simulink model "five_bar_model_discrete_v_0"  (R2018a)
settings: Solver=ode45  StartTime=0.0  StopTime=tmax  FixedStep=0.0001  MaxStep=1e-3  RelTol=1e-3
values from neighbouring files (symbols this model uses):
  dt = 10e-3    (= 0.01)    [model_parameters_v_1.m]    (also in test_dynamics.m = 0.2; test_kinematics.m = 0.1)
  g = -9.80665    [idyn5.m]    (also in test_dynamics.m; test_model.m = 9.80665)
  Kd = (3*aj*wj-Fv) * eye(2)    [model_parameters_v_1.m]
  Kdi = [2 * zita *  wpos1; 2  * zita * wpos2]    [model_parameters_v_1.m]
  Ki = aj*wj^3 * eye(2)    [model_parameters_v_1.m]
  Kp = 3*aj*wj^2 * eye(2)    [model_parameters_v_1.m]
  Kpi = [ wpos1^2;  wpos2^2]    [model_parameters_v_1.m]
  p = [NaN; NaN]    [fkine5.m]    (also in test_model.m = zeros(n,2))
  p0 = p(:,1)    [model_parameters_v_1.m]    (also in test_dynamics.m = [x(i);y(i)]; test_kinematics.m = [0; 0.35])
  q = [NaN; NaN; NaN; NaN; NaN]    [fkine5.m]    (also in ikine5.m = [q11;q12;q13;q21;q22])
  q0 = q(:,1)    [model_parameters_v_1.m]    (also in test_dynamics.m = q0(:,4); test_kinematics.m = q0(:,4))
  qd = [qda(1);qdu(1);qdu(2);qda(2);qdu(3)]    [ifirstkine5.m]
  qdd = [qdda(1);qddu(1);qddu(2);qdda(2);qddu(3)]    [isecondkine5.m]
  t0r = J * qda    [ffirstkine5.m]    (also in test_dynamics.m = [0;0]; test_kinematics.m = [1;1]; test_model.m = p)
  t0r0 = t0r(:,1)    [model_parameters_v_1.m]
  t0rd = (J * qdda+ at)    [fsecondkine5.m]    (also in test_dynamics.m = [0;0]; test_kinematics.m = [-1;1]; test_model.m = p)
  t0rd0 = t0rd(:,1)    [model_parameters_v_1.m]
undefined symbols (not defined in the file or in its folder): DiscIntNeverNeededParam, Kii, tmax, X, Y, Z
libraries: sm_lib x24, simulink x16, nesl_utility x9, powerlib_meascontrol x1
(part 3 of 3)

== matlab function five_bar_model_discrete_v_0/five-bar-robot2/forward kinematics ==
  data: qa input; p output; assembly input; q output
function [p,q] = fkine5(qa, assembly)
% This function implement the forward kinematic model of a five bar robot
% @parm qa: active joint positions vector 2x1
% @parm assembly: assembly mode selecction 1 for + -1 for -
% @return p: p end-effector coordinate vector 2X1
% @return q: joint positon vector 5X1
    l = 0.205;
    d1 = [-0.125, l, l];
    d2 = [0.125, l, l];
    q11 = qa(1);
    q21 = qa(2);

    A12 = [d1(2)*cos(q11)+d1(1); d1(2)*sin(q11)];
    A22 = [d2(2)*cos(q21)+d2(1); d2(2)*sin(q21)];

    if sqrt((A12-A22)' * (A12-A22)) <= 2*l
        a1 = - 2*d1(1) - 2*d1(2)*cos(q11);
        a2 = - 2*d2(1) - 2*d2(2)*cos(q21);
        b1 = - 2*sin(q11)*d1(2);
        b2 = - 2*sin(q21)*d2(2);
        c1 = d1(1)^2 + 2*cos(q11)*d1(1)*d1(2) + d1(2)^2 - d1(3)^2;
        c2 = d2(1)^2 + 2*cos(q21)*d2(1)*d2(2) + d2(2)^2 - d2(3)^2;

        if b1 ~= b2
            a = a2 - a1;
            b = b2 - b1;
            c = c2 - c1;
            e1 = - a / b;
            e2 = - c / b;
            f1 = 1 + e1^2;
            f2 = 2 * e1 * e2 + a1 + b1 * e1;
            f3 = e2^2 + b1 * e2 + c1;

            x = (-f2 - sqrt(f2^2 - 4 * f1 * f3)) / (2 * f1);
            y = e1 * x + e2;

            A13=[x-A12(1);y-A12(2)];
            A23=[x-A22(1);y-A22(2)];
            if  A13(1)*A23(2)-A23(1)*A13(2) <= 0 && assembly == 1
                x = (-f2 + sqrt(f2^2 - 4 * f1 * f3)) / (2 * f1);
                y = e1 * x + e2;
            elseif  A13(1)*A23(2)-A23(1)*A13(2) >= 0 && assembly == -1
                x = (-f2 + sqrt(f2^2 - 4 * f1 * f3)) / (2 * f1);
                y = e1 * x + e2;
            end
        else
            x = - (c2 - c1) / (a2 - a1);
            y = (-b1 + (b1^2 - 4 * (x^2 + a1 * x + c1))^(1/2)) / 2;

            A13=[x-A12(1);y-A12(2)];
            A23=[x-A22(1);y-A22(2)];
            if  A13(1)*A23(2)-A23(1)*A13(2) <= 0 && assembly == 1
                y = (-b1 - (b1^2 - 4 * (x^2 + a1 * x + c1))^(1/2)) / 2;
            elseif  A13(1)*A23(2)-A23(1)*A13(2) >= 0 && assembly == -1
                y = (-b1 - (b1^2 - 4 * (x^2 + a1 * x + c1))^(1/2)) / 2;
            end
        end

        % for q12 and q22 from a12/a11 and a22/a21
        q12 = atan2(y-d1(2)*sin(q11), x-d1(1)-d1(2)*cos(q11)) - q11;
        q22 = atan2(y-d2(2)*sin(q21), x-d2(1)-d2(2)*cos(q21)) - q21;
        q13 = q21 + q22 - q11 - q12;
        p = [x;y];
        q = [q11; q12; q13; q21; q22];
        
        % I will work in the first assembly.
        % Note: A way of implement the change of assembly is using the equations
        % (3) and (4) of the paper Minimum-time trajectory planning and control
        % of a pick-and-place five-bar parallel robot. Obtaining the
        % previous assembly, then the current and finally comparing
        % eache other.
%         sum(angdiff(q, q_prev).^2)
%         if sum(angdiff(q, q_prev).^2) > 0.1 
%             disp('Atention!!');
%             assembly2 = -assembly;
%             q11 = qa(1);
%             q21 = qa(2);
%             a1 = - 2*d1(1) - 2*d1(2)*cos(q11);
%             a2 = - 2*d2(1) - 2*d2(2)*cos(q21);
%             b1 = - 2*sin(q11)*d1(2);
%             b2 = - 2*sin(q21)*d2(2);
%             c1 = d1(1)^2 + 2*cos(q11)*d1(1)*d1(2) + d1(2)^2 - d1(3)^2;
%             c2 = d2(1)^2 + 2*cos(q21)*d2(1)*d2(2) + d2(2)^2 - d2(3)^2;
% 
%             if b1 ~= b2
%                 a = a2 - a1;
%                 b = b2 - b1;
%                 c = c2 - c1;
%                 e1 = - a / b;
%                 e2 = - c / b;
%                 f1 = 1 + e1^2;
%                 f2 = 2 * e1 * e2 + a1 + b1 * e1;
%                 f3 = e2^2 + b1 * e2 + c1;
% 
%                 x = (-f2 - sqrt(f2^2 - 4 * f1 * f3)) / (2 * f1);
%                 y = e1 * x + e2;
% 
%                 A13=[x-A12(1);y-A12(2)];
%                 A23=[x-A22(1);y-A22(2)];
%                 if  A13(1)*A23(2)-A23(1)*A13(2) <= 0 && assembly2 == 1
%                     x = (-f2 + sqrt(f2^2 - 4 * f1 * f3)) / (2 * f1);
%                     y = e1 * x + e2;
%                 elseif  A13(1)*A23(2)-A23(1)*A13(2) >= 0 && assembly2 == -1
%                     x = (-f2 + sqrt(f2^2 - 4 * f1 * f3)) / (2 * f1);
%                     y = e1 * x + e2;
%                 end
%             else
%                 x = - (c2 - c1) / (a2 - a1);
%                 y = (-b1 + (b1^2 - 4 * (x^2 + a1 * x + c1))^(1/2)) / 2;
% 
%                 A13=[x-A12(1);y-A12(2)];
%                 A23=[x-A22(1);y-A22(2)];
%                 if  A13(1)*A23(2)-A23(1)*A13(2) <= 0 && assembly == 1
%                     y = (-b1 - (b1^2 - 4 * (x^2 + a1 * x + c1))^(1/2)) / 2;
%                 elseif  A13(1)*A23(2)-A23(1)*A13(2) >= 0 && assembly == -1
%                     y = (-b1 - (b1^2 - 4 * (x^2 + a1 * x + c1))^(1/2)) / 2;
%                 end
%             end
% 
%             % for q12 and q22 from a12/a11 and a22/a21
%             q12 = atan2(y-d1(2)*sin(q11), x-d1(1)-d1(2)*cos(q11)) - q11;
%             q22 = atan2(y-d2(2)*sin(q21), x-d2(1)-d2(2)*cos(q21)) - q21;
%             q13 = q21 + q22 - q11 - q12;
%             p = [x;y];
%             q = [q11; q12; q13; q21; q22];
%         end
    else
        disp('ERROR: Euclidian distance > 2*l');
        p = [NaN; NaN];
        q = [NaN; NaN; NaN; NaN; NaN];
    end

== matlab function five_bar_model_discrete_v_0/five-bar-robot2/inverse dynamics ==
  data: q input; T output double size=2; qd input; qdd input; t0rd input; J input; Jt input; Jta input; Jtd input; Psit input
function T  = idyn5(q,qd,qdd,t0rd,J,Jt,Jta,Jtd,Psit)

    l = 0.205;
    d1 = [-0.125, l, l];
    d2 = [0.125, l, l];
    q1 = q(1:3);
    q2 = q(4:5);
    qd1 = qd(1:3);
    qd2 = qd(4:5);
    qdd1 = qdd(1:3);
    qdd2 = qdd(4:5);
    xdd = t0rd(1);
    ydd = t0rd(2);
    Tt1 = zeros(3,1);
    Tt2 = zeros(2,1);
    Ttd = zeros(3,1);
    % Dynamic
    % Gravity 
%     g = -9.80665;
    g = 0;
% Dynamics parameters
    m11 = 0.126; %kg
    mx11 = m11 * 0.1025;
    my11 =  0; %m11 * 1.44e-2;
    zz11 = 0.001774; %kg-m^2;
    
    m12 = 0.126; %kg
    mx12 = m12 * 0.1025;
    my12 =  0; %m11 * 1.44e-2;
    zz12 = 0.001774; %kg-m^2;
    
    m21 = 0.126; %kg
    mx21 = m21 * 0.1025;
    my21 =  0; %m11 * 1.44e-2;
    zz21 = 0.001774; %kg-m^2;
    
    m22 = 0.126; %kg
    mx22 = m22 * 0.1025;
    my22 =  0; %m11 * 1.44e-2;
    zz22 = 0.001774; %kg-m^2;
    
    Ia11 = 4.8e-5; % kg-m2
%     zz11r = zz11 + Ia11 + d1(2)^2 * m12;
    
    Ia21 = 4.8e-5; % kg-m2
%     zz21r = zz21 + Ia21 + d2(2)^2 * m22;
   
    %Fricciones fv = viscosa fs= seca
    fv1 = [1.5e-1 0 0];
    fs1 = [1.5e-1 0 0];
    fv2 = [0 0];
    fs2 = [0 0];
    % End effector mass
    m4 = 0.272;

    % Inverse dynamics model
    Tt1(1) = (my12*sin(q1(1) + q1(2)) - mx12*cos(q1(1) + q1(2)) ...
        - mx11*cos(q1(1)) + my11*sin(q1(1)) - d1(2)*m12*cos(q1(1)))*g ...
        + Ia11*qdd1(1) + fv1(1)*qd1(1) + fs1(1)*sign(qd1(1)) ...
        + mx12*(- d1(2)*sin(q1(2))*qd1(2)^2 - 2*d1(2)*qd1(1)*sin(q1(2))*qd1(2) ...
        + 2*d1(2)*qdd1(1)*cos(q1(2)) + d1(2)*qdd1(2)*cos(q1(2))) ...
        - my12*(d1(2)*cos(q1(2))*qd1(2)^2 + 2*d1(2)*qd1(1)*cos(q1(2))*qd1(2) ...
        + 2*d1(2)*qdd1(1)*sin(q1(2)) + d1(2)*qdd1(2)*sin(q1(2))) ...
        + qdd1(1)*zz11 + qdd1(1)*zz12 + qdd1(2)*zz12 + m12*qdd1(1)*d1(2)^2;
    Tt1(2) = (my12*sin(q1(1) + q1(2)) - mx12*cos(q1(1) + q1(2)))*g ...
        + zz12*(qdd1(1) + qdd1(2)) + fv1(2)*qd1(2) + fs1(2)*sign(qd1(2)) ...
        + mx12*(d1(2)*sin(q1(2))*qd1(1)^2 + d1(2)*qdd1(1)*cos(q1(2))) ...
        - my12*(-d1(2)*cos(q1(2))*qd1(1)^2 + d1(2)*qdd1(1)*sin(q1(2)));
    Tt1(3) = fs1(3) * sign(qd1(3)) + fv1(3)*qd1(3);
    
    Tt2(1) = (my22*sin(q2(1) + q2(2)) - mx22*cos(q2(1) + q2(2)) ...
        - mx21*cos(q2(1)) + my21*sin(q2(1)) - d2(2)*m22*cos(q2(1)))*g ...
        + Ia21*qdd2(1) + fv2(1)*qd2(1) + fs2(1)*sign(qd2(1)) ...
        + mx22*(- d2(2)*sin(q2(2))*qd2(2)^2 - 2*d2(2)*qd2(1)*sin(q2(2))*qd2(2) ...
        + 2*d2(2)*qdd2(1)*cos(q2(2)) + d2(2)*qdd2(2)*cos(q2(2))) ...
        - my22*(d2(2)*cos(q2(2))*qd2(2)^2 + 2*d2(2)*qd2(1)*cos(q2(2))*qd2(2) ...
        + 2*d2(2)*qdd2(1)*sin(q2(2)) + d2(2)*qdd2(2)*sin(q2(2))) ...
        + qdd2(1)*zz21 + qdd2(1)*zz22 + qdd2(2)*zz22 + m22*qdd2(1)*d2(2)^2;
   
    Tt2(2) = (my22*sin(q2(1) + q2(2)) - mx22*cos(q2(1) + q2(2)))*g ...
        + zz22*(qdd2(1) + qdd2(2)) + fv2(2)*qd2(2) + fs2(2)*sign(qd2(2)) ...
        + mx22*(d2(2)*sin(q2(2))*qd2(1)^2 + d2(2)*qdd2(1)*cos(q2(2))) ...
        - my22*(-d2(2)*cos(q2(2))*qd2(1)^2 + d2(2)*qdd2(1)*sin(q2(2)));

    % End effector like a punctual mass fixed on B22
    w0p = m4 * [xdd; ydd-g; zeros(4,1)];
    w0r = Psit' * w0p;
    % IDM
    Tta = [Tt1(1); Tt2(1)];
    Ttd = [Tt1(2:3); Tt2(2)];

    Jd = (Jtd) \ (Jt * J - Jta);

    T = Tta + J' * w0r + Jd' * Ttd;

== matlab function five_bar_model_discrete_v_0/five-bar-robot2/inverse kinematics ==
  data: p input; q output; q_prev input; qa output; qp output; stop output boolean
function [q,qa,qp,stop] = ikine5(p, q_prev)
% This function implement the inverse kinematic model of a five bar robot
% @parm p: p end-effector coordinate vector 2X1
% @parm q_prev: previos joint position vector 5X1
% @return q: joint positions vector 5x1
% @return qa: active joints positions vector 2X1
% @return qp: underactuated joints positions vector 3X1

    l = 0.205;
    d11 = -0.125;
    d12 = l;
    d13 = l;
    d21 = 0.125;
    d22 = l;
    d23 = l;
    x = p(1);
    y = p(2);
    q_aux = zeros(5,4);

    dist013 = sqrt((p(1)-d11)^2+p(2)^2);
    dist023 = sqrt((p(1)-d21)^2+p(2)^2);
    if dist013 <= 2*l && dist023 <= 2*l
        % q11 = -2*atan((((d11^2 - 2*d11*x - d12^2 + 2*d12*d13 - d13^2 + x^2 + y^2)*(- d11^2 + 2*d11*x + d12^2 + 2*d12*d13 + d13^2 - x^2 - y^2))^(1/2) - 2*d12*y)/(d11^2 - 2*d11*d12 - 2*d11*x + d12^2 + 2*d12*x - d13^2 + x^2 + y^2));
        a1 = -2*d12*(x-d11);
        b1 = -2*d12*y;
        c1 = (x-d11)^2+y^2+d12^2-d13^2;
        q11 = 2*atan((-b1-sqrt(b1^2-c1^2+a1^2)) / (c1-a1));
        if ~isreal(q11)
            q_aux(:,1) = [NaN, NaN, NaN, NaN, NaN]';
            q_aux(:,2) = [NaN, NaN, NaN, NaN, NaN]';
        else
            % q21 = -2*atan((((d21^2 - 2*d21*x - d22^2 + 2*d22*d23 - d23^2 + x^2 + y^2)*(- d21^2 + 2*d21*x + d22^2 + 2*d22*d23 + d23^2 - x^2 - y^2))^(1/2) - 2*d22*y)/(d21^2 - 2*d21*d22 - 2*d21*x + d22^2 + 2*d22*x - d23^2 + x^2 + y^2));
            a2 = -2*d22*(x-d21);
            b2 = -2*d22*y;
            c2 = (x-d21)^2+y^2+d22^2-d23^2;
            q21 = 2*atan((-b2+sqrt(b2^2-c2^2+a2^2)) /(c2-a2));
            if ~isreal(q21)
                q_aux(:,1) = [NaN, NaN, NaN, NaN, NaN]';
            else
                q12 = - q11 + atan2(y - d12*sin(q11), x - d11 - d12*cos(q11));
                q22 = - q21 + atan2(y - d22*sin(q21), x - d21 - d22*cos(q21));
                q13 = q21 - q12 - q11 + q22;
                q_aux(:,1) = [q11, q12, q13, q21, q22]';
            end
            % q21 = 2*atan((((d21^2 - 2*d21*x - d22^2 + 2*d22*d23 - d23^2 + x^2 + y^2)*(- d21^2 + 2*d21*x + d22^2 + 2*d22*d23 + d23^2 - x^2 - y^2))^(1/2) + 2*d22*y)/(d21^2 - 2*d21*d22 - 2*d21*x + d22^2 + 2*d22*x - d23^2 + x^2 + y^2));
            q21 = 2*atan((-b2-sqrt(b2^2-c2^2+a2^2)) /(c2-a2));
            if ~isreal(q21)
                q_aux(:,2) = [NaN, NaN, NaN, NaN, NaN]';
            else
                q12 = - q11 + atan2(y - d12*sin(q11), x - d11 - d12*cos(q11));
                q22 = - q21 + atan2(y - d22*sin(q21), x - d21 - d22*cos(q21));
                q13 = q21 - q12 - q11 + q22;
                q_aux(:,2) = [q11, q12, q13, q21, q22]';
            end
        end

        % q11 = 2*atan((((d11^2 - 2*d11*x - d12^2 + 2*d12*d13 - d13^2 + x^2 + y^2)*(- d11^2 + 2*d11*x + d12^2 + 2*d12*d13 + d13^2 - x^2 - y^2))^(1/2) + 2*d12*y)/(d11^2 - 2*d11*d12 - 2*d11*x + d12^2 + 2*d12*x - d13^2 + x^2 + y^2));
        q11 = 2*atan((-b1+sqrt(b1^2-c1^2+a1^2)) / (c1-a1));
        if ~isreal(q11)
            q_aux(:,3) = [NaN, NaN, NaN, NaN, NaN]';
            q_aux(:,4) = [NaN, NaN, NaN, NaN, NaN]';
        else
            % q21 = -2*atan((((d21^2 - 2*d21*x - d22^2 + 2*d22*d23 - d23^2 + x^2 + y^2)*(- d21^2 + 2*d21*x + d22^2 + 2*d22*d23 + d23^2 - x^2 - y^2))^(1/2) - 2*d22*y)/(d21^2 - 2*d21*d22 - 2*d21*x + d22^2 + 2*d22*x - d23^2 + x^2 + y^2));
            q21 = 2*atan((-b2+sqrt(b2^2-c2^2+a2^2)) /(c2-a2));
            if ~isreal(q21)
                q_aux(:,3) = [NaN, NaN, NaN, NaN, NaN]';
            else
                q12 = - q11 + atan2(y - d12*sin(q11), x - d11 - d12*cos(q11));
                q22 = - q21 + atan2(y - d22*sin(q21), x - d21 - d22*cos(q21));
                q13 = q21 - q12 - q11 + q22;
                q_aux(:,3) = [q11, q12, q13, q21, q22]';
            end
            % q21 = 2*atan((((d21^2 - 2*d21*x - d22^2 + 2*d22*d23 - d23^2 + x^2 + y^2)*(- d21^2 + 2*d21*x + d22^2 + 2*d22*d23 + d23^2 - x^2 - y^2))^(1/2) + 2*d22*y)/(d21^2 - 2*d21*d22 - 2*d21*x + d22^2 + 2*d22*x - d23^2 + x^2 + y^2));
            q21 = 2*atan((-b2-sqrt(b2^2-c2^2+a2^2)) /(c2-a2));
            if ~isreal(q21)
                q_aux(:,4) = [NaN, NaN, NaN, NaN, NaN]';
            else
                q12 = - q11 + atan2(y - d12*sin(q11), x - d11 - d12*cos(q11));
                q22 = - q21 + atan2(y - d22*sin(q21), x - d21 - d22*cos(q21));
                q13 = q21 - q12 - q11 + q22;
                q_aux(:,4) = [q11, q12, q13, q21, q22]';
            end
        end
        % find the correct working mode base in the previous mode
        % qa(:,i) = [q(1,3);q(4,3)]; 
        if nargin < 2
            q = q_aux; %(:,1);
            qa = [q(1,:); q(4,:)];
            qp = [q(2:3,:); q(5,:)];
        else
            distance_between_q = sum(angdiff(q_aux, q_prev * ones(1,4)).^2);
            index = find(distance_between_q == min(distance_between_q));
            q = q_aux(:,index(1));
            qa = [q(1); q(4)];
            qp = [q(2:3); q(5)];
        end
        stop = false;
    else
        disp('ERROR: point out of work space');
%             q = [NaN; NaN; NaN; NaN; NaN];
            q = q_prev;
            stop = true;
            qa = [q(1); q(4)];
            qp = [q(2:3); q(5)];
        % point out of work space
    end

== matlab function five_bar_model_discrete_v_0/five-bar-robot2/scond order forward kinematic ==
  data: qdda input; t0rd output; qd input; q input; Ar input; J input
function t0rd  = fsecondkine5(qdda,qd,q,Ar,J)
% This function implement the second-order forward kinematics model of a five bar robot
% @param qdda: active acceleration joints vector 2X1
% @param qd: velocity joints vector 5x1
% @param q: joint positions vector 5x1
% @param Ar: matrix 2x2 for computation of the dynamic model of the PKM
% @param J: kinematic Jacobian matrix of the PKM
% @return t0rd: derivate twist end-effector vector 2X1
    l = 0.205;
    d1 = [-0.125, l, l];
    d2 = [0.125, l, l];
    q1 = q(1:3);
    q2 = q(4:5);
    qd1 = qd(1:3);
    qd2 = qd(4:5);

    wr1 = [cos(q1(1)+q1(2)); sin(q1(1)+q1(2)); 0; 0; 0; 0];
    wr2 = [cos(q2(1)+q2(2)); sin(q2(1)+q2(2)); 0; 0; 0; 0];

    b01a_ = [-d1(2)*qd1(1)*cos(q1(1)) - d1(3)*cos(q1(1)+q1(2))*(qd1(1)+qd1(2));
             -d1(2)*qd1(1)*sin(q1(1)) - d1(3)*sin(q1(1)+q1(2))*(qd1(1)+qd1(2));
             zeros(4,1)];
    b01b_ = [-d1(3)*cos(q1(1)+q1(2));
             -d1(3)*sin(q1(1)+q1(2));
             zeros(4,1)];
    b0p1 = b01a_ * qd1(1) + b01b_ * qd1(2)*(qd1(1)+qd1(2));

    b02a_ = [-d2(2)*qd2(1)*cos(q2(1)) - d2(3)*cos(q2(1)+q2(2))*(qd2(1)+qd2(2));
             -d2(2)*qd2(1)*sin(q2(1)) - d2(3)*sin(q2(1)+q2(2))*(qd2(1)+qd2(2));
             zeros(4,1)];
    b02b_ = [-d2(3)*cos(q2(1)+q2(2));
             -d2(3)*sin(q2(1)+q2(2));
             zeros(4,1)];
    b0p2 = b02a_ * qd2(1) + b02b_ * qd2(2)*(qd2(1)+qd2(2));

    b0p = [(wr1'*b0p1); (wr2'*b0p2)];

    at = pinv(Ar) * b0p;
    t0rd = (J * qdda + at);

== matlab function five_bar_model_discrete_v_0/five-bar-robot2/second order inverse kinematics ==
  data: t0rd input; qdd output; t0r input; p input; q input; qd input; Ar input; B input; Jinv input; Jt input; Jta input; Jtd input; Psit input; qdda output; qddu output; Psit1 output; Psit2 output; atp output; ad output
function [qdd,qdda,qddu,Psit1,Psit2,atp,ad] = isecondkine5(t0rd,t0r,p,q,qd,Ar,B,Jinv,Jt,Jta,Jtd,Psit)
% This function implement the second-order inverse kinematics model of a five bar robot
% @param t0rd: derivate twist end-effector vector 2X1
% @param t0r: twist end-effector vector 2X1
% @param p: end-effector coordinate vector 2X1
% @param q: joint positions vector 5x1
% @param qd: velocity joints vector 5x1
% @param Ar: matrix 2x2 for computation of the dynamic model of the PKM
% @param B: matrix 2x2 for computation of the dynamic model of the PKM
% @param Jinv: inverse kinematic Jacobian matrix of the PKM
% @param Jt: crucial for computation of the dynamic model of the PKM.
% @param Jta: crucial for computation of the dynamic model of the PKM.
% @param Jtd: crucial for computation of the dynamic model of the PKM.
% @return qdd: acceleration joint vector 5x1
% @return qdda: active acceleration joints vector 2X1
% @return qddu: underactuated acceleration joints vector 3X1
% @return Psit1: matrix 2x6
% @return Psit2: matrix 1x6
% @return atp: acceleration using for dynamics
% @return ad: acceleration using for dynamics

    l = 0.205;
    d1 = [-0.125, l, l];
    d2 = [0.125, l, l];
    q1 = q(1:3);
    q2 = q(4:5);
    qd1 = qd(1:3);
    qd2 = qd(4:5);
    Phi = sum(q1);
    Phid = sum(qd1);
    x = p(1);
    y = p(2);
    xd = t0r(1);
    yd = t0r(2);

    wr1 = [cos(q1(1)+q1(2)); sin(q1(1)+q1(2)); 0; 0; 0; 0];
    wr2 = [cos(q2(1)+q2(2)); sin(q2(1)+q2(2)); 0; 0; 0; 0];

    b01a_ = [-d1(2)*qd1(1)*cos(q1(1)) - d1(3)*cos(q1(1)+q1(2))*(qd1(1)+qd1(2));
             -d1(2)*qd1(1)*sin(q1(1)) - d1(3)*sin(q1(1)+q1(2))*(qd1(1)+qd1(2));
             zeros(4,1)];
    b01b_ = [-d1(3)*cos(q1(1)+q1(2));
             -d1(3)*sin(q1(1)+q1(2));
             zeros(4,1)];
    b0p1 = b01a_ * qd1(1) + b01b_ * qd1(2)*(qd1(1)+qd1(2));

    b02a_ = [-d2(2)*qd2(1)*cos(q2(1)) - d2(3)*cos(q2(1)+q2(2))*(qd2(1)+qd2(2));
             -d2(2)*qd2(1)*sin(q2(1)) - d2(3)*sin(q2(1)+q2(2))*(qd2(1)+qd2(2));
             zeros(4,1)];
    b02b_ = [-d2(3)*cos(q2(1)+q2(2));
             -d2(3)*sin(q2(1)+q2(2));
             zeros(4,1)];
    b0p2 = b02a_ * qd2(1) + b02b_ * qd2(2)*(qd2(1)+qd2(2));

    b0p = [(wr1'*b0p1); (wr2'*b0p2)];

    aqq = pinv(B) * b0p;
    qdda = (Jinv * t0rd + aqq);

    % Aceleracion pasiva

    ayd = (Phid*sin(2*Phi))/(d2(1) - x + d2(2)*cos(q2(1))) - (cos(Phi)^2*(xd + d2(2)*qd2(1)*sin(q2(1))))/(d2(1) - x + d2(2)*cos(q2(1)))^2;

    axd = (Phid*sin(2*Phi)*(y - d2(2)*sin(q2(1))))/(d2(1) - x + d2(2)*cos(q2(1)))^2 ...
        - (cos(Phi)^2*(yd - d2(2)*qd2(1)*cos(q2(1))))/(d2(1) - x + d2(2)*cos(q2(1)))^2 ...
        - (2*cos(Phi)^2*(xd + d2(2)*qd2(1)*sin(q2(1)))*(y - d2(2)*sin(q2(1))))/(d2(1) - x + d2(2)*cos(q2(1)))^3;

    aqd = (2*d2(2)*cos(Phi)^2*(xd + d2(2)*qd2(1)*sin(q2(1)))*(d2(2) - sin(q2(1))*y + cos(q2(1))*(d2(1) - x)))...
        /(d2(1) - x + d2(2)*cos(q2(1)))^3 ...
        - (d2(2)*cos(Phi)^2*(xd*cos(q2(1)) + yd*sin(q2(1)) + qd2(1)*cos(q2(1))*y + qd2(1)*sin(q2(1))*(d2(1) - x)))...
        /(d2(1) - x + d2(2)*cos(q2(1)))^2 ...
        - (2*Phid*d2(2)*cos(Phi)*sin(Phi)*(d2(2) - sin(q2(1))*y + cos(q2(1))*(d2(1) - x)))...
        /(d2(1) - x + d2(2)*cos(q2(1)))^2;

    j21_invd = -(sin(q2(1) + q2(2))*(qd2(1) + qd2(2)))/(d2(2)*sin(q2(2))) ...
               -(qd2(2)*cos(q2(1) + q2(2))*cos(q2(2)))/(d2(2)*sin(q2(2))^2);

    j22_invd = -(qd2(2)*sin(q2(1) + q2(2))*cos(q2(2)))/(d2(2)*sin(q2(2))^2) ...
               +(cos(q2(1) + q2(2))*(qd2(1) + qd2(2)))/(d2(2)*sin(q2(2)));

    aq = -(d2(2) * ((x-d2(1))*cos(q2(1))+y*sin(q2(1))-d2(2))*cos(Phi)^2) / (x - d2(2)*cos(q2(1)) - d2(1))^2;

    psitd1 = axd + aqd*Jinv(2,1)+ aq*j21_invd;
    psitd2 = ayd + aqd*Jinv(2,2)+ aq*j22_invd;

    Psidt = [0 0; 0 0; 0 0; 0 0; 0 0; psitd1 psitd2];

    Psit1 = [-sin(q1(1)+q1(2)) cos(q1(1)+q1(2)) 0 0 0 0
             0                 0                0 0 0 1];
    Psit2 = [-sin(q2(1)+q2(2)) cos(q2(1)+q2(2)) 0 0 0 0];

    dc1 = Psit1 * (eye(6)* Psidt * t0r - b0p1); % Jti = I6x6 -> di = 06x1
    dc2 = Psit2 * (eye(6)* Psidt * t0r - b0p2);
    dc = [dc1;
          dc2];

    qddu =  Jtd\(Jt*t0rd - Jta*qdda + dc);

    qdd = [qdda(1);qddu(1);qddu(2);qdda(2);qddu(3)];

    at = pinv(Ar) * b0p;
    atp = Psit * at + Psidt * t0r;% using for dynamics
    ad = Jtd \ (dc + Jt*at); % For dynamics
